simulink model "test_core"  (R2016b)
settings: Solver=VariableStepAuto  StartTime=0.0  StopTime=10000  RelTol=1e-3
values from neighbouring files (symbols this model uses):
  a_b = 1.656E-05    (= 1.656e-05)    [Parameters_Core_PHE.m]    (also in Parameters_Core_PHE_FEHE.m; Parameters_MSBR.m; Parameters_MSBR_Brayton.m; Parameters_MSBR_new_nodal.m)
  A_Bgn = A_Bg/nn_Bg    [Parameters_MSBR_new_nodal.m]    (also in Parameters_steady_state.m)
  a_f = -8.172E-05    (= -8.172e-05)    [Parameters_Core_PHE.m]    (also in Parameters_Core_PHE_FEHE.m; Parameters_MSBR.m; Parameters_MSBR_Brayton.m; Parameters_MSBR_new_nodal.m)
  A_fgboren = A_fgbore/nn_fdn    (= 52.5696341877)    [Parameters_MSBR_new_nodal.m]    (also in Parameters_steady_state.m)
  A_fgsleidn = A_fgsleid/nn_fup    (= 29.0039361035)    [Parameters_MSBR_new_nodal.m]    (also in Parameters_steady_state.m)
  A_fgsleodn = A_fgsleod/nn_fdn    (= 43.5059041553)    [Parameters_MSBR_new_nodal.m]    (also in Parameters_steady_state.m)
  a_g = 2.016E-05    (= 2.016e-05)    [Parameters_Core_PHE.m]    (also in Parameters_Core_PHE_FEHE.m; Parameters_MSBR.m; Parameters_MSBR_Brayton.m; Parameters_MSBR_new_nodal.m)
  A_ggin = A_ggi/nn_gg    [Parameters_MSBR_new_nodal.m]    (also in Parameters_steady_state.m)
  A_ggon = A_ggo/nn_gg    [Parameters_MSBR_new_nodal.m]    (also in Parameters_steady_state.m)
  beta = [2.290E-04, 8.320E-04, 7.100E-04, 8.520E-04, 1.710E-04, 1.020E-04]    [Parameters_Core_PHE.m]    (also in Parameters_Core_PHE_FEHE.m; Parameters_MSBR.m; Parameters_MSBR_Brayton.m; Parameters_MSBR_new_nodal.m)
  beta_t = sum(beta)    [Parameters_Core_PHE.m]    (also in Parameters_Core_PHE_FEHE.m; Parameters_MSBR.m; Parameters_MSBR_Brayton.m; Parameters_MSBR_new_nodal.m)
  C0 = lam.\beta/Lam    [parameters_msbr_pke_stat.m]
  Cp_B = 9.207E-04    (= 0.0009207)    [Parameters_MSBR_new_nodal.m]    (also in Parameters_steady_state.m = 0.0009211)
  Cp_f = 2.302E-03    (= 0.002302)    [Parameters_MSBR_new_nodal.m]    (also in Parameters_steady_state.m)
  Cp_g = 1.679E-03    (= 0.001679)    [Parameters_MSBR_new_nodal.m]    (also in Parameters_steady_state.m)
  h_Bg = 2.839E-03    (= 0.002839)    [Parameters_MSBR_new_nodal.m]    (also in Parameters_steady_state.m)
  h_fgi = 9.176E-03    (= 0.009176)    [Parameters_MSBR_new_nodal.m]    (also in Parameters_steady_state.m)
  h_fgo = 8.165E-03    (= 0.008165)    [Parameters_MSBR_new_nodal.m]    (also in Parameters_steady_state.m)
  h_ggi = cond_g/l_i    [Parameters_MSBR_new_nodal.m]    (also in Parameters_steady_state.m)
  h_ggo = cond_g/l_o    [Parameters_MSBR_new_nodal.m]    (also in Parameters_steady_state.m)
  k_Ba1 = 8.500E-03/2    (= 0.00425)    [Parameters_MSBR_new_nodal.m]    (also in Parameters_steady_state.m)
  k_Ba2 = 8.500E-03/2    (= 0.00425)    [Parameters_MSBR_new_nodal.m]    (also in Parameters_steady_state.m)
  k_Bb1 = 8.500E-03/2    (= 0.00425)    [Parameters_MSBR_new_nodal.m]    (also in Parameters_steady_state.m)
  k_Bb2 = 8.500E-03/2    (= 0.00425)    [Parameters_MSBR_new_nodal.m]    (also in Parameters_steady_state.m)
  k_BL = 1-k_core    [Parameters_MSBR_new_nodal.m]    (also in Parameters_steady_state.m)
  k_f1a1 = 2.210E-01/2    (= 0.1105)    [Parameters_MSBR_new_nodal.m]    (also in Parameters_steady_state.m)
  k_f1a2 = 2.210E-01/2    (= 0.1105)    [Parameters_MSBR_new_nodal.m]    (also in Parameters_steady_state.m)
  k_f1b1 = 2.210E-01/2    (= 0.1105)    [Parameters_MSBR_new_nodal.m]    (also in Parameters_steady_state.m)
  k_f1b2 = 2.210E-01/2    (= 0.1105)    [Parameters_MSBR_new_nodal.m]    (also in Parameters_steady_state.m)
  k_f2a1 = 2.210E-01/2    (= 0.1105)    [Parameters_MSBR_new_nodal.m]    (also in Parameters_steady_state.m)
  k_f2a2 = 2.210E-01/2    (= 0.1105)    [Parameters_MSBR_new_nodal.m]    (also in Parameters_steady_state.m)
  k_f2b1 = 2.210E-01/2    (= 0.1105)    [Parameters_MSBR_new_nodal.m]    (also in Parameters_steady_state.m)
  k_f2b2 = 2.210E-01/2    (= 0.1105)    [Parameters_MSBR_new_nodal.m]    (also in Parameters_steady_state.m)
  k_g1a = rkmf*m_g1a    [Parameters_MSBR_new_nodal.m]    (also in Parameters_steady_state.m)
  k_g1b = rkmf*m_g1b    [Parameters_MSBR_new_nodal.m]    (also in Parameters_steady_state.m)
  k_g2a = rkmf*m_g2a    [Parameters_MSBR_new_nodal.m]    (also in Parameters_steady_state.m)
  k_g2b = rkmf*m_g2b    [Parameters_MSBR_new_nodal.m]    (also in Parameters_steady_state.m)
  k_g3a = rkmf*m_g3a    [Parameters_MSBR_new_nodal.m]    (also in Parameters_steady_state.m)
  k_g3b = rkmf*m_g3b    [Parameters_MSBR_new_nodal.m]    (also in Parameters_steady_state.m)
  k_g4a = (rkmB*m_gB+rkmf*(m_g4a+m_g4b-m_gB))/2    [Parameters_MSBR_new_nodal.m]    (also in Parameters_steady_state.m)
  k_g4b = (rkmB*m_gB+rkmf*(m_g4a+m_g4b-m_gB))/2    [Parameters_MSBR_new_nodal.m]    (also in Parameters_steady_state.m)
  Lam = 3.300E-04    (= 0.00033)    [Parameters_Core_PHE.m]    (also in Parameters_Core_PHE_FEHE.m; Parameters_MSBR.m; Parameters_MSBR_Brayton.m; Parameters_MSBR_new_nodal.m)
  lam = [0.0126,0.0337,0.139,0.325,1.13,2.50]'    [PKE_general.m]    (also in Parameters_Core_PHE.m = [1.260E-02, 3.370E-02, 1.390E-01, 3.250E-01, 1.130E+00, 2.50; Parameters_Core_PHE_FEHE.m = [1.260E-02, 3.370E-02, 1.390E-01, 3.250E-01, 1.130E+00, 2.50; Parameters_MSBR.m = [1.260E-02, 3.370E-02, 1.390E-01, 3.250E-01, 1.130E+00, 2.50; Parameters_MSBR_Brayton.m = [1.260E-02, 3.370E-02, 1.390E-01, 3.250E-01, 1.130E+00, 2.50)
  m_Ba1 = m_B/nn_B    (= 941.25)    [Parameters_MSBR_new_nodal.m]    (also in Parameters_steady_state.m = 2092.75)
  m_Ba2 = m_B/nn_B    (= 941.25)    [Parameters_MSBR_new_nodal.m]    (also in Parameters_steady_state.m = 2092.75)
  m_Bb1 = m_B/nn_B    (= 941.25)    [Parameters_MSBR_new_nodal.m]    (also in Parameters_steady_state.m = 2092.75)
  m_Bb2 = m_B/nn_B    (= 941.25)    [Parameters_MSBR_new_nodal.m]    (also in Parameters_steady_state.m = 2092.75)
  m_BL = k_BL*m_B/(k_Bb1+k_Bb2+k_Ba1+k_Ba2)    [Parameters_MSBR_new_nodal.m]    (also in Parameters_steady_state.m = 22804.35)
  m_Bm = W_B    (= 269)    [Parameters_MSBR_new_nodal.m]    (also in Parameters_steady_state.m = 271.65)
  m_f1a1 = mn_f    (= 597)    [Parameters_MSBR_new_nodal.m]    (also in Parameters_steady_state.m = 1004.5)
  m_f1a2 = mn_f    (= 597)    [Parameters_MSBR_new_nodal.m]    (also in Parameters_steady_state.m = 1004.5)
  m_f1b1 = mn_f    (= 597)    [Parameters_MSBR_new_nodal.m]    (also in Parameters_steady_state.m = 1004.5)
  m_f1b2 = mn_f    (= 597)    [Parameters_MSBR_new_nodal.m]    (also in Parameters_steady_state.m = 1004.5)
  m_f2a1 = mn_f    (= 597)    [Parameters_MSBR_new_nodal.m]    (also in Parameters_steady_state.m = 1004.5)
  m_f2a2 = mn_f    (= 597)    [Parameters_MSBR_new_nodal.m]    (also in Parameters_steady_state.m = 1004.5)
  m_f2b1 = mn_f    (= 597)    [Parameters_MSBR_new_nodal.m]    (also in Parameters_steady_state.m = 1004.5)
  m_f2b2 = mn_f    (= 597)    [Parameters_MSBR_new_nodal.m]    (also in Parameters_steady_state.m = 1004.5)
  m_g1a = rho_g*(pi*r_msle^2 - pi*(sle_ID/2)^2)*l_cell*n_cell/2    [Parameters_MSBR_new_nodal.m]    (also in Parameters_steady_state.m = (rho_g*(pi*r_msle^2 - pi*(sle_ID/2)^2)*l_cell*n_cell/2))
  m_g1b = rho_g*(pi*r_msle^2 - pi*(sle_ID/2)^2)*l_cell*n_cell/2    [Parameters_MSBR_new_nodal.m]    (also in Parameters_steady_state.m = (rho_g*(pi*r_msle^2 - pi*(sle_ID/2)^2)*l_cell*n_cell/2))
  m_g2a = rho_g*(pi*(sle_OD/2)^2 - pi*r_msle^2)*l_cell*n_cell/2    [Parameters_MSBR_new_nodal.m]    (also in Parameters_steady_state.m = (rho_g*(pi*(sle_OD/2)^2 - pi*r_msle^2)*l_cell*n_cell/2))
  m_g2b = rho_g*(pi*(sle_OD/2)^2 - pi*r_msle^2)*l_cell*n_cell/2    [Parameters_MSBR_new_nodal.m]    (also in Parameters_steady_state.m = (rho_g*(pi*(sle_OD/2)^2 - pi*r_msle^2)*l_cell*n_cell/2))
  m_g3a = rho_g*(pi*r_mhex^2 - pi*(bore_OD/2)^2)*l_cell*n_cell/2    [Parameters_MSBR_new_nodal.m]    (also in Parameters_steady_state.m = (rho_g*(pi*r_mhex^2 - pi*(bore_OD/2)^2)*l_cell*n_cell/2))
  m_g3b = rho_g*(pi*r_mhex^2 - pi*(bore_OD/2)^2)*l_cell*n_cell/2    [Parameters_MSBR_new_nodal.m]    (also in Parameters_steady_state.m = (rho_g*(pi*r_mhex^2 - pi*(bore_OD/2)^2)*l_cell*n_cell/2))
  m_g4a = rho_g*(A_hex - pi*r_mhex^2)*l_cell*n_cell/2    [Parameters_MSBR_new_nodal.m]    (also in Parameters_steady_state.m = (rho_g*(A_hex - pi*r_mhex^2)*l_cell*n_cell/2))
  m_g4b = rho_g*(A_hex - pi*r_mhex^2)*l_cell*n_cell/2    [Parameters_MSBR_new_nodal.m]    (also in Parameters_steady_state.m = (rho_g*(A_hex - pi*r_mhex^2)*l_cell*n_cell/2))
  n_frac0 = 1    [Parameters_Core_PHE.m]    (also in Parameters_Core_PHE_FEHE.m; Parameters_MSBR.m; Parameters_MSBR_Brayton.m; Parameters_MSBR_new_nodal.m)
  P = 556.0    (= 556)    [Parameters_Core_PHE.m]    (also in Parameters_Core_PHE_FEHE.m; Parameters_MSBR.m; Parameters_MSBR_Brayton.m; Parameters_MSBR_new_nodal.m)
  T0_Ba1 = T0_b2-(T0_b2-T_b_in)*(1/4)    (= 662.7725)    [Parameters_MSBR_new_nodal.m]    (also in Parameters_steady_state.m)
  T0_Ba2 = T0_b2    (= 676.66)    [Parameters_MSBR_new_nodal.m]    (also in Parameters_steady_state.m)
  T0_Bb1 = T0_b2-(T0_b2-T_b_in)*(3/4)    (= 634.9975)    [Parameters_MSBR_new_nodal.m]    (also in Parameters_steady_state.m)
  T0_Bb2 = T0_b2-(T0_b2-T_b_in)*(2/4)    (= 648.885)    [Parameters_MSBR_new_nodal.m]    (also in Parameters_steady_state.m)
  T0_BL = T0_Ba2    (= 676.66)    [Parameters_MSBR_new_nodal.m]    (also in Parameters_steady_state.m)
  T0_f1a1 = T0_f4-(T0_f4-Tf_in)*(2/8)    (= 662.7725)    [Parameters_MSBR_new_nodal.m]    (also in Parameters_steady_state.m)
  T0_f1a2 = T0_f4-(T0_f4-Tf_in)*(3/8)    (= 641.93875)    [Parameters_MSBR_new_nodal.m]    (also in Parameters_steady_state.m)
  T0_f1b1 = T0_f4    (= 704.44)    [Parameters_MSBR_new_nodal.m]    (also in Parameters_steady_state.m)
  T0_f1b2 = T0_f4-(T0_f4-Tf_in)*(1/8)    (= 683.60625)    [Parameters_MSBR_new_nodal.m]    (also in Parameters_steady_state.m)
  T0_f2a1 = T0_f4-(T0_f4-Tf_in)*(4/8)    (= 621.105)    [Parameters_MSBR_new_nodal.m]    (also in Parameters_steady_state.m)
  T0_f2a2 = T0_f4-(T0_f4-Tf_in)*(5/8)    (= 600.27125)    [Parameters_MSBR_new_nodal.m]    (also in Parameters_steady_state.m)
  T0_f2b1 = T0_f4-(T0_f4-Tf_in)*(6/8)    (= 579.4375)    [Parameters_MSBR_new_nodal.m]    (also in Parameters_steady_state.m)
  T0_f2b2 = T0_f4-(T0_f4-Tf_in)*(7/8)    (= 558.60375)    [Parameters_MSBR_new_nodal.m]    (also in Parameters_steady_state.m)
  T0_g1a = (A+B*T0_f1a2+C/E*(A+D+B*T0_f1a2+E*T0_f2a2))/(B+C+B*C/E)    [Parameters_MSBR_new_nodal.m]    (also in Parameters_steady_state.m = (2*A*(C+E) + 4*B*(C+E)*T0_f1a2 + 2*C*E*T0_f2a2 - 2*C*B*T0_f1)
  T0_g1b = (A+B*T0_f1b2+C/E*(A+D+B*T0_f1b2+E*T0_f2b2))/(B+C+B*C/E)    [Parameters_MSBR_new_nodal.m]    (also in Parameters_steady_state.m = (2*A*(C+E) + 4*B*(C+E)*T0_f1b2 + 2*C*E*T0_f2b2 - 2*C*B*T0_f1)
  T0_g2a = (A+D+B*T0_f1a2-B*T0_g1a+E*T0_f2a2)/E    [Parameters_MSBR_new_nodal.m]    (also in Parameters_steady_state.m = (2*E*T0_f2a2 + 2*B*(T0_g1a - T0_f1a2))/(2*(C+E)))
  T0_g2b = (A+D+B*T0_f1b2-B*T0_g1b+E*T0_f2b2)/E    [Parameters_MSBR_new_nodal.m]    (also in Parameters_steady_state.m = (2*E*T0_f2b2 + 2*B*(T0_g1b - T0_f1b2))/(2*(C+E)))
  T0_g3a = (F+G*T0_f2a2+H/J*(F+I+G*T0_f2a2+J*T0_Ba1))/(G+H+G*H/J)    [Parameters_MSBR_new_nodal.m]    (also in Parameters_steady_state.m = (2*F*(H+J) + 4*G*(H+J)*T0_f2a2 + 2*H*J*T0_Ba1 - 2*H*G*T0_f2a)
  T0_g3b = (F+G*T0_f2b2+H/J*(F+I+G*T0_f2b2+J*T0_Bb1))/(G+H+G*H/J)    [Parameters_MSBR_new_nodal.m]    (also in Parameters_steady_state.m = (2*F*(H+J) + 4*G*(H+J)*T0_f2b2 + 2*H*J*T0_Bb1 - 2*H*G*T0_f2b)
  T0_g4a = (F+I+G*T0_f2a2-G*T0_g3a+J*T0_Ba1)/J    [Parameters_MSBR_new_nodal.m]    (also in Parameters_steady_state.m = (2*J*T0_Ba1 + 2*G*(T0_g3a - T0_f2a2))/(2*(H+J)))
  T0_g4b = (F+I+G*T0_f2b2-G*T0_g3b+J*T0_Bb1)/J    [Parameters_MSBR_new_nodal.m]    (also in Parameters_steady_state.m = (2*J*T0_Bb1 + 2*G*(T0_g3b - T0_f2b2))/(2*(H+J)))
  T_b_in = 621.11    [Parameters_Core_PHE.m]    (also in Parameters_Core_PHE_FEHE.m; Parameters_MSBR.m; Parameters_MSBR_Brayton.m; Parameters_MSBR_new_nodal.m)
  tau_c = 3.28    [Parameters_Core_PHE.m]    (also in Parameters_Core_PHE_FEHE.m; Parameters_MSBR.m; Parameters_MSBR_Brayton.m; Parameters_MSBR_new_nodal.m)
  tau_l = 5.85    [Parameters_Core_PHE.m]    (also in Parameters_Core_PHE_FEHE.m; Parameters_MSBR.m; Parameters_MSBR_Brayton.m; Parameters_MSBR_new_nodal.m)
  Tf_in = 537.77    [Parameters_Core_PHE.m]    (also in Parameters_Core_PHE_FEHE.m; Parameters_MSBR.m; Parameters_MSBR_Brayton.m; Parameters_MSBR_new_nodal.m)
  W_B = 2.690E+02    (= 269)    [Parameters_MSBR_new_nodal.m]    (also in Parameters_steady_state.m = 271.65)
  W_BL = m_BL*W_B/m_B    [Parameters_MSBR_new_nodal.m]    (also in Parameters_steady_state.m = 270.14)
  W_f = 1.414E3    (= 1414)    [Parameters_Core_PHE.m]    (also in Parameters_Core_PHE_FEHE.m; Parameters_MSBR.m; Parameters_MSBR_Brayton.m; Parameters_MSBR_new_nodal.m)
settings Model: Creator=mlish  LastModifiedBy=mlish

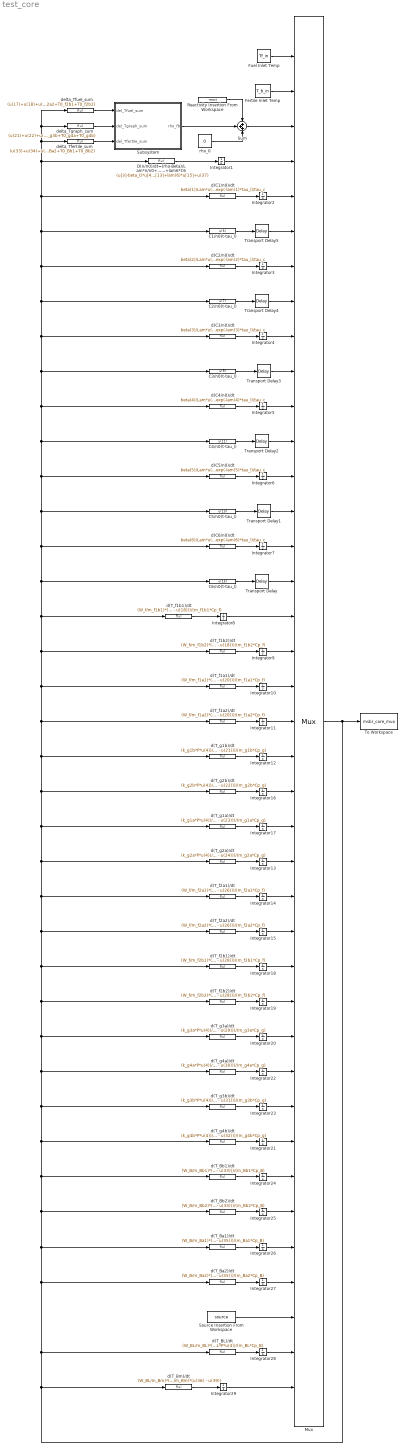
== system test_core ==
  C1/n0(t-tau_l) : Fcn  Expr=u(5)
  C2/n0(t-tau_l) : Fcn  Expr=u(7)
  C3/n0(t-tau_l) : Fcn  Expr=u(9)
  C4/n0(t-tau_l) : Fcn  Expr=u(11)
  C5/n0(t-tau_l) : Fcn  Expr=u(13)
  C6/n0(t-tau_l) : Fcn  Expr=u(15)
  D(n/n0)/dt=(rho-Beta)/Lam*n/n0+lam1*C1+...+lam6*C6 : Fcn  Expr=(u[3]-beta_t)*u[4]/Lam+lam(1)*u[5]+lam(2)*u[7]+lam(3)*u[9]+lam(4)*u[11]+lam(5)*u[13]+lam(6)*u[15]+u(37)
  Fertile Inlet Temp : Constant  Value=T_b_in
  Fuel Inlet Temp : Constant  Value=Tf_in
  Integrator1 : Integrator  InitialCondition=n_frac0
  Integrator10 : Integrator  InitialCondition=T0_f1a1
  Integrator11 : Integrator  InitialCondition=T0_f1a2
  Integrator12 : Integrator  InitialCondition=T0_g1b
  Integrator13 : Integrator  InitialCondition=T0_g2a
  Integrator14 : Integrator  InitialCondition=T0_f2a1
  Integrator15 : Integrator  InitialCondition=T0_f2a2
  Integrator16 : Integrator  InitialCondition=T0_g2b
  Integrator17 : Integrator  InitialCondition=T0_g1a
  Integrator18 : Integrator  InitialCondition=T0_f2b1
  Integrator19 : Integrator  InitialCondition=T0_f2b2
  Integrator2 : Integrator  InitialCondition=C0(1)
  Integrator20 : Integrator  InitialCondition=T0_g3a
  Integrator21 : Integrator  InitialCondition=T0_g4b
  Integrator22 : Integrator  InitialCondition=T0_g4a
  Integrator23 : Integrator  InitialCondition=T0_g3b
  Integrator24 : Integrator  InitialCondition=T0_Bb1
  Integrator25 : Integrator  InitialCondition=T0_Bb2
  Integrator26 : Integrator  InitialCondition=T0_Ba1
  Integrator27 : Integrator  InitialCondition=T0_Ba2
  Integrator28 : Integrator  InitialCondition=T0_BL
  Integrator29 : Integrator  InitialCondition=T0_BL
  Integrator3 : Integrator  InitialCondition=C0(2)
  Integrator4 : Integrator  InitialCondition=C0(3)
  Integrator5 : Integrator  InitialCondition=C0(4)
  Integrator6 : Integrator  InitialCondition=C0(5)
  Integrator7 : Integrator  InitialCondition=C0(6)
  Integrator8 : Integrator  InitialCondition=T0_f1b1
  Integrator9 : Integrator  InitialCondition=T0_f1b2
  Mux : Mux  Inputs=39
      settings: DisplayOption=signals
  Reactivity Insertion From Workspace : FromWorkspace  VariableName=react  SampleTime=1  Interpolate=off  OutputAfterFinalValue=Holding final value
  Source Insertion From Workspace : FromWorkspace  VariableName=source  SampleTime=1  Interpolate=off  OutputAfterFinalValue=Holding final value
  Subsystem : Subsystem
  Sum : Sum  Inputs=+++
  To Workspace : ToWorkspace  VariableName=msbr_core_mux  SampleTime=-1
  Transport Delay : TransportDelay  DelayTime=tau_l  InitialOutput=C0(6)  BufferSize=4096
  Transport Delay1 : TransportDelay  DelayTime=tau_l  InitialOutput=C0(5)  BufferSize=4096
  Transport Delay2 : TransportDelay  DelayTime=tau_l  InitialOutput=C0(4)  BufferSize=4096
  Transport Delay3 : TransportDelay  DelayTime=tau_l  InitialOutput=C0(3)  BufferSize=4096
  Transport Delay4 : TransportDelay  DelayTime=tau_l  InitialOutput=C0(2)  BufferSize=4096
  Transport Delay5 : TransportDelay  DelayTime=tau_l  InitialOutput=C0(1)  BufferSize=4096
  d(C1/n0)/dt : Fcn  Expr=beta(1)/Lam*u(4)-lam(1)*u(5)-u(5)/tau_c+u(6)*exp(-lam(1)*tau_l)/tau_c
  d(C2/n0)/dt : Fcn  Expr=beta(2)/Lam*u(4)-lam(2)*u(7)-u(7)/tau_c+u(8)*exp(-lam(2)*tau_l)/tau_c
  d(C3/n0)/dt : Fcn  Expr=beta(3)/Lam*u(4)-lam(3)*u(9)-u(9)/tau_c+u(10)*exp(-lam(3)*tau_l)/tau_c
  d(C4/n0)/dt : Fcn  Expr=beta(4)/Lam*u(4)-lam(4)*u(11)-u(11)/tau_c+u(12)*exp(-lam(4)*tau_l)/tau_c
  d(C5/n0)/dt : Fcn  Expr=beta(5)/Lam*u(4)-lam(5)*u(13)-u(13)/tau_c+u(14)*exp(-lam(5)*tau_l)/tau_c
  d(C6/n0)/dt : Fcn  Expr=beta(6)/Lam*u(4)-lam(6)*u(15)-u(15)/tau_c+u(16)*exp(-lam(6)*tau_l)/tau_c
  d(T_BL)/dt : Fcn  Expr=(W_BL/m_BL)*(u(2) - u(38)) + (k_BL*P*u(4))/(m_BL*Cp_B)
  d(T_Ba1)/dt : Fcn  Expr=(W_B/m_Ba1)*(u(34) - u(35)) + (k_Ba1*P*u(4))/(m_Ba1*Cp_B) + (h_Bg*A_Bgn*(u(30) - u(35)))/(m_Ba1*Cp_B)
  d(T_Ba2)/dt : Fcn  Expr=(W_B/m_Ba2)*(u(35) - u(36)) + (k_Ba2*P*u(4))/(m_Ba2*Cp_B) + (h_Bg*A_Bgn*(u(30) - u(35)))/(m_Ba2*Cp_B)
  d(T_Bb1)/dt : Fcn  Expr=(W_B/m_Bb1)*(u(2) - u(33)) + (k_Bb1*P*u(4))/(m_Bb1*Cp_B) + (h_Bg*A_Bgn*(u(32) - u(33)))/(m_Bb1*Cp_B)
  d(T_Bb2)/dt : Fcn  Expr=(W_B/m_Bb2)*(u(33) - u(34)) + (k_Bb2*P*u(4))/(m_Bb2*Cp_B) + (h_Bg*A_Bgn*(u(32) - u(33)))/(m_Bb2*Cp_B)
  d(T_Bm)/dt : Fcn  Expr=(W_BL/m_Bm)*(u(38) - u(39)) + (W_B/m_Bm)*(u(36) - u(39))
  d(T_f1a1)/dt : Fcn  Expr=(W_f/m_f1a1)*(u(20) - u(19)) + (k_f1a1*P*u(4))/(m_f1a1*Cp_f) + (h_fgi*A_fgsleidn*(u(23) - u(20)))/(m_f1a1*Cp_f)
  d(T_f1a2)/dt : Fcn  Expr=(W_f/m_f1a2)*(u(25) - u(20)) + (k_f1a2*P*u(4))/(m_f1a2*Cp_f) + (h_fgi*A_fgsleidn*(u(23) - u(20)))/(m_f1a2*Cp_f)
  d(T_f1b1)/dt : Fcn  Expr=(W_f/m_f1b1)*(u(18) - u(17)) + (k_f1b1*P*u(4))/(m_f1b1*Cp_f) + (h_fgi*A_fgsleidn*(u(21) - u(18)))/(m_f1b1*Cp_f)
  d(T_f1b2)/dt : Fcn  Expr=(W_f/m_f1b2)*(u(19) - u(18)) + (k_f1b2*P*u(4))/(m_f1b2*Cp_f) + (h_fgi*A_fgsleidn*(u(21) - u(18)))/(m_f1b2*Cp_f)
  d(T_f2a1)/dt : Fcn  Expr=(W_f/m_f2a1)*(u(26) - u(25)) + (k_f2a1*P*u(4))/(m_f2a1*Cp_f) + (h_fgo*A_fgsleodn*(u(24) - u(26)))/(m_f2a1*Cp_f) + (h_fgo*A_fgboren*(u(29) - u(26)))/(m_f2a1*Cp_f)
  d(T_f2a2)/dt : Fcn  Expr=(W_f/m_f2a2)*(u(27) - u(26)) + (k_f2a2*P*u(4))/(m_f2a2*Cp_f) + (h_fgo*A_fgsleodn*(u(24) - u(26)))/(m_f2a2*Cp_f) + (h_fgo*A_fgboren*(u(29) - u(26)))/(m_f2a2*Cp_f)
  d(T_f2b1)/dt : Fcn  Expr=(W_f/m_f2b1)*(u(28) - u(27)) + (k_f2b1*P*u(4))/(m_f2b1*Cp_f) + (h_fgo*A_fgsleodn*(u(22) - u(28)))/(m_f2b1*Cp_f) + (h_fgo*A_fgboren*(u(31) - u(28)))/(m_f2b1*Cp_f)
  d(T_f2b2)/dt : Fcn  Expr=(W_f/m_f2b2)*(u(1) - u(28)) + (k_f2b2*P*u(4))/(m_f2b2*Cp_f) + (h_fgo*A_fgsleodn*(u(22) - u(28)))/(m_f2b2*Cp_f) + (h_fgo*A_fgboren*(u(31) - u(28)))/(m_f2b2*Cp_f)
  d(T_g1a)/dt : Fcn  Expr=(k_g1a*P*u(4))/(m_g1a*Cp_g) + (2*h_fgi*A_fgsleidn*(u(20) - u(23)))/(m_g1a*Cp_g) + (h_ggi*A_ggin*(u(24) - u(23)))/(m_g1a*Cp_g)
  d(T_g1b)/dt : Fcn  Expr=(k_g1b*P*u(4))/(m_g1b*Cp_g) + (2*h_fgi*A_fgsleidn*(u(18) - u(21)))/(m_g1b*Cp_g) + (h_ggi*A_ggin*(u(22) - u(21)))/(m_g1b*Cp_g)
  d(T_g2a)/dt : Fcn  Expr=(k_g2a*P*u(4))/(m_g2a*Cp_g) + (2*h_fgo*A_fgsleodn*(u(26) - u(24)))/(m_g2a*Cp_g) + (h_ggi*A_ggin*(u(23) - u(24)))/(m_g2a*Cp_g)
  d(T_g2b)/dt : Fcn  Expr=(k_g2b*P*u(4))/(m_g2b*Cp_g) + (2*h_fgo*A_fgsleodn*(u(28) - u(22)))/(m_g2b*Cp_g) + (h_ggi*A_ggin*(u(21) - u(22)))/(m_g2b*Cp_g)
  d(T_g3a)/dt : Fcn  Expr=(k_g3a*P*u(4))/(m_g3a*Cp_g) + (2*h_fgo*A_fgboren*(u(26) - u(29)))/(m_g3a*Cp_g) + (h_ggo*A_ggon*(u(30) - u(29)))/(m_g3a*Cp_g)
  d(T_g3b)/dt : Fcn  Expr=(k_g3b*P*u(4))/(m_g3b*Cp_g) + (2*h_fgo*A_fgboren*(u(28) - u(31)))/(m_g3b*Cp_g) + (h_ggo*A_ggon*(u(32) - u(31)))/(m_g3b*Cp_g)
  d(T_g4a)/dt : Fcn  Expr=(k_g4a*P*u(4))/(m_g4a*Cp_g) + (2*h_Bg*A_Bgn*(u(35) - u(30)))/(m_g4a*Cp_g) + (h_ggo*A_ggon*(u(29) - u(30)))/(m_g4a*Cp_g)
  d(T_g4b)/dt : Fcn  Expr=(k_g4b*P*u(4))/(m_g4b*Cp_g) + (2*h_Bg*A_Bgn*(u(33) - u(32)))/(m_g4b*Cp_g) + (h_ggo*A_ggon*(u(31) - u(32)))/(m_g4b*Cp_g)
  delta_Tfertile_sum : Fcn  Expr=(u(33)+u(34)+u(35)+u(36)) - (T0_Ba1+T0_Ba2+T0_Bb1+T0_Bb2)
  delta_Tfuel_sum : Fcn  Expr=(u(17)+u(18)+u(19)+u(20)+u(25)+u(26)+u(27)+u(28)) - (T0_f1a1+T0_f1a2+T0_f1b1+T0_f1b2+T0_f2a1+T0_f2a2+T0_f2b1+T0_f2b2)
  delta_Tgraph_sum : Fcn  Expr=(u(21)+u(22)+u(23)+u(24)+u(29)+u(30)+u(31)+u(32)) - (T0_g1a+T0_g1b+T0_g2a+T0_g2b+T0_g3a+T0_g3b+T0_g4a+T0_g4b)
  rho_0 : Constant  Value=0
  wires:
  d(T_f1b1)/dt/1 -> Integrator8/1
  d(T_f1b2)/dt/1 -> Integrator9/1
  d(T_f1a1)/dt/1 -> Integrator10/1
  d(T_f1a2)/dt/1 -> Integrator11/1
  d(T_g1b)/dt/1 -> Integrator12/1
  Integrator12/1 -> Mux/21
  Integrator11/1 -> Mux/20
  Integrator10/1 -> Mux/19
  Integrator9/1 -> Mux/18
  Integrator8/1 -> Mux/17
  D(n/n0)/dt=(rho-Beta)/Lam*n/n0+lam1*C1+...+lam6*C6/1 -> Integrator1/1
  d(C1/n0)/dt/1 -> Integrator2/1
  d(C2/n0)/dt/1 -> Integrator3/1
  d(C3/n0)/dt/1 -> Integrator4/1
  d(C4/n0)/dt/1 -> Integrator5/1
  d(C5/n0)/dt/1 -> Integrator6/1
  d(C6/n0)/dt/1 -> Integrator7/1
  Integrator1/1 -> Mux/4
  Integrator2/1 -> Mux/5
  Integrator3/1 -> Mux/7
  Integrator4/1 -> Mux/9
  Integrator5/1 -> Mux/11
  Integrator6/1 -> Mux/13
  Integrator7/1 -> Mux/15
  C6/n0(t-tau_l)/1 -> Transport Delay/1
  Transport Delay/1 -> Mux/16
  C5/n0(t-tau_l)/1 -> Transport Delay1/1
  Transport Delay1/1 -> Mux/14
  Transport Delay2/1 -> Mux/12
  C4/n0(t-tau_l)/1 -> Transport Delay2/1
  C3/n0(t-tau_l)/1 -> Transport Delay3/1
  Transport Delay3/1 -> Mux/10
  Transport Delay4/1 -> Mux/8
  C2/n0(t-tau_l)/1 -> Transport Delay4/1
  Transport Delay5/1 -> Mux/6
  C1/n0(t-tau_l)/1 -> Transport Delay5/1
  Sum/1 -> Mux/3
  Reactivity Insertion From Workspace/1 -> Sum/1
  delta_Tfuel_sum/1 -> Subsystem/1(del_Tfuel_sum)
  delta_Tgraph_sum/1 -> Subsystem/2(del_Tgraph_sum)
  delta_Tfertile_sum/1 -> Subsystem/3(del_Tfertile_sum)
  Subsystem/1(rho_fb) -> Sum/2
  Source Insertion From Workspace/1 -> Mux/37
  d(T_g2b)/dt/1 -> Integrator16/1
  d(T_g1a)/dt/1 -> Integrator17/1
  d(T_g2a)/dt/1 -> Integrator13/1
  d(T_f2a1)/dt/1 -> Integrator14/1
  d(T_f2a2)/dt/1 -> Integrator15/1
  Integrator15/1 -> Mux/26
  Integrator14/1 -> Mux/25
  Integrator13/1 -> Mux/24
  Integrator17/1 -> Mux/23
  Integrator16/1 -> Mux/22
  d(T_f2b1)/dt/1 -> Integrator18/1
  d(T_f2b2)/dt/1 -> Integrator19/1
  Integrator18/1 -> Mux/27
  d(T_g3a)/dt/1 -> Integrator20/1
  Integrator20/1 -> Mux/29
  d(T_g4a)/dt/1 -> Integrator22/1
  d(T_g3b)/dt/1 -> Integrator23/1
  d(T_g4b)/dt/1 -> Integrator21/1
  Integrator21/1 -> Mux/32
  Integrator23/1 -> Mux/31
  Integrator22/1 -> Mux/30
  d(T_Bb1)/dt/1 -> Integrator24/1
  d(T_Bb2)/dt/1 -> Integrator25/1
  Integrator25/1 -> Mux/34
  Integrator24/1 -> Mux/33
  d(T_Ba1)/dt/1 -> Integrator26/1
  d(T_Ba2)/dt/1 -> Integrator27/1
  Integrator27/1 -> Mux/36
  Integrator26/1 -> Mux/35
  Mux/1 -> d(T_Bm)/dt/1, d(T_BL)/dt/1, d(T_Ba2)/dt/1, d(T_Ba1)/dt/1, d(T_Bb2)/dt/1, d(T_Bb1)/dt/1, d(T_g4b)/dt/1, d(T_g3b)/dt/1, d(T_g4a)/dt/1, d(T_g3a)/dt/1, d(T_f2b2)/dt/1, d(T_f2b1)/dt/1, d(T_f2a2)/dt/1, d(T_f2a1)/dt/1, d(T_g2a)/dt/1, d(T_g1a)/dt/1, d(T_g2b)/dt/1, delta_Tfertile_sum/1, delta_Tgraph_sum/1, delta_Tfuel_sum/1, D(n/n0)/dt=(rho-Beta)/Lam*n/n0+lam1*C1+...+lam6*C6/1, d(C1/n0)/dt/1, C1/n0(t-tau_l)/1, d(C2/n0)/dt/1, C2/n0(t-tau_l)/1, d(C3/n0)/dt/1, C3/n0(t-tau_l)/1, d(C4/n0)/dt/1, C4/n0(t-tau_l)/1, d(C5/n0)/dt/1, C5/n0(t-tau_l)/1, d(C6/n0)/dt/1, C6/n0(t-tau_l)/1, d(T_f1b1)/dt/1, d(T_f1b2)/dt/1, d(T_f1a1)/dt/1, d(T_f1a2)/dt/1, d(T_g1b)/dt/1, To Workspace/1
  Integrator19/1 -> Mux/28
  d(T_BL)/dt/1 -> Integrator28/1
  Integrator28/1 -> Mux/38
  d(T_Bm)/dt/1 -> Integrator29/1
  Integrator29/1 -> Mux/39
  Fuel Inlet Temp/1 -> Mux/1
  Fertile Inlet Temp/1 -> Mux/2
  rho_0/1 -> Sum/3

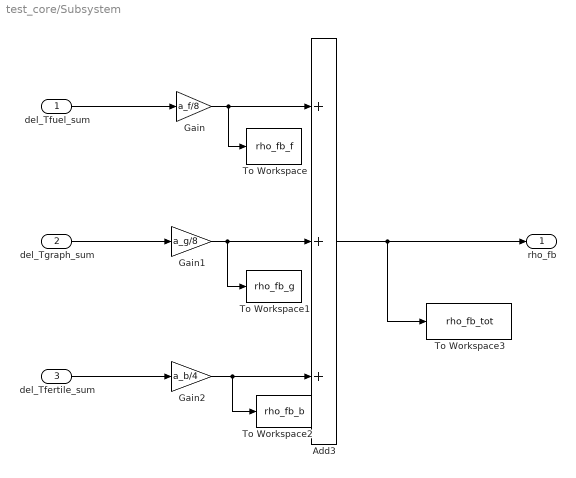
== system test_core/Subsystem ==
  del_Tfuel_sum : Inport
  del_Tgraph_sum : Inport  Port=2
  del_Tfertile_sum : Inport  Port=3
  Add3 : Sum  Inputs=+++
  Gain : Gain  Gain=a_f/8
  Gain1 : Gain  Gain=a_g/8
  Gain2 : Gain  Gain=a_b/4
  To Workspace : ToWorkspace  VariableName=rho_fb_f  SampleTime=-1
  To Workspace1 : ToWorkspace  VariableName=rho_fb_g  SampleTime=-1
  To Workspace2 : ToWorkspace  VariableName=rho_fb_b  SampleTime=-1
  To Workspace3 : ToWorkspace  VariableName=rho_fb_tot  SampleTime=-1
  rho_fb : Outport
  wires:
  del_Tfuel_sum/1 -> Gain/1
  del_Tgraph_sum/1 -> Gain1/1
  del_Tfertile_sum/1 -> Gain2/1
  Gain1/1 -> To Workspace1/1, Add3/2
  Gain/1 -> To Workspace/1, Add3/1
  Add3/1 -> To Workspace3/1, rho_fb/1
  Gain2/1 -> To Workspace2/1, Add3/3
